simulink model "mikti_sim"  (R2023a)
settings: Solver=ode23tb  StartTime=0.0  StopTime=15  MaxStep=1e-5  MinStep=1e-5  RelTol=1e-4
values from neighbouring files (symbols this model uses):
  A = 0:-1:-50    [mikti.m]
  l = A(i)    [mikti.m]
libraries: spsSeriesRLCBranchLib x9, spsControlledCurrentSourceLib x2, spsCurrentMeasurementLib x2, spsDCVoltageSourceLib x1, spsDCMachineLib x1, spsVoltageMeasurementLib x1, spsControlledVoltageSourceLib x1, sps_lib x1
settings Model: Creator=User  LastModifiedBy=gpapa
settings SolverCC: AlgebraicLoopSolver=TrustRegion
settings DataIOCC: ReturnWorkspaceOutputs=off
settings DebuggingCC: UnconnectedInputMsg=warning  UnconnectedOutputMsg=warning  UnconnectedLineMsg=warning  ArithmeticOperatorsInVariantConditions=warning
settings ModelReferenceCC: EnableRefExpFcnMdlSchedulingChecks=on
settings SFSimCC: CustomCodeUndefinedFunction=UseInterfaceOnly

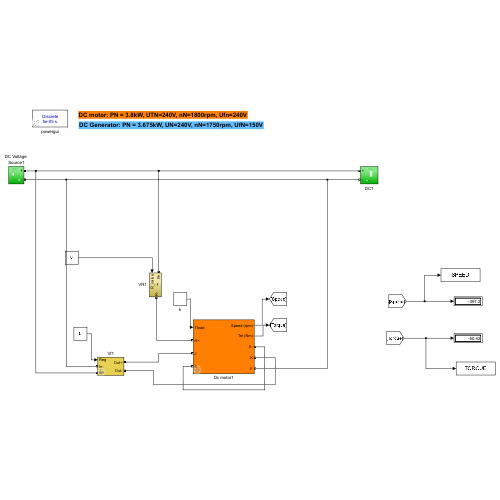
[thumbnail: Simulink's stored preview of the top-level diagram]
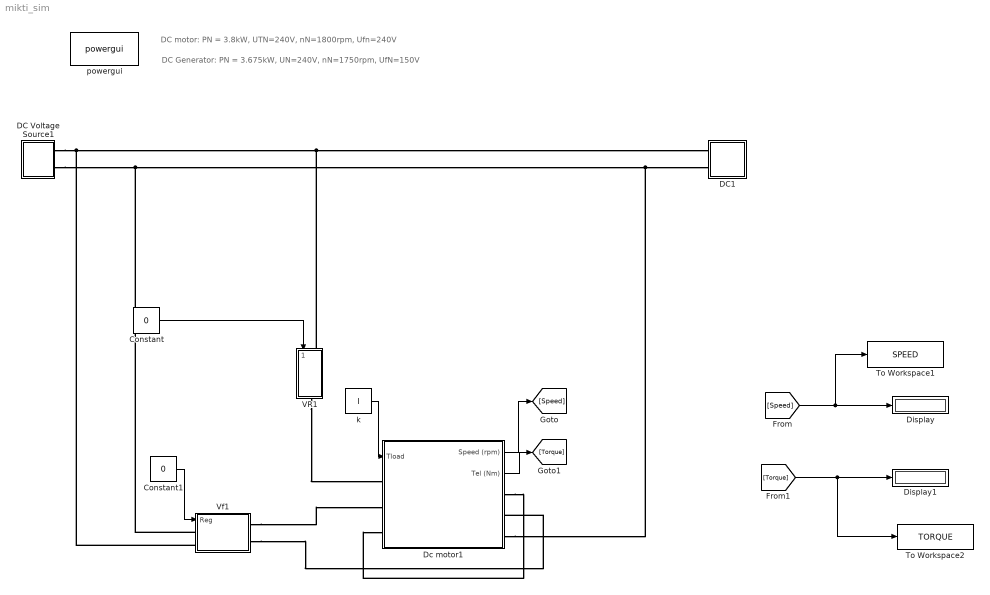
== system mikti_sim ==
  note: DC motor: PN = 3.8kW, UTN=240V, nN=1800rpm, Ufn=240V
  note: DC Generator: PN = 3.675kW, UN=240V, nN=1750rpm, UfN=150V
  Constant : Constant  Value=0
  Constant1 : Constant  Value=0
  DC Voltage Source1 : Subsystem
  DC1 : Subsystem
  Dc motor1 : Subsystem  mask{PN=3.8, VN=240, nN=1800}
      mask prompts: PN "PN (kW)"; VN "VN (V)"; nN "nN (rpm)"
      mask DialogControl Control2 Prompt: DC Motor
  Display : Display
  Display1 : Display
  To Workspace1 : ToWorkspace  VariableName=SPEED  SaveFormat=Structure With Time  SampleTime=-1
      settings: MaxDataPoints=1
  To Workspace2 : ToWorkspace  VariableName=TORQUE  SaveFormat=Structure With Time  SampleTime=-1
      settings: MaxDataPoints=1
  VR1 : Subsystem
  Vf1 : Subsystem  mask{R=230}
      mask prompts: R "R (Ω)"
      mask DialogControl Label1 Prompt: Variable Resistor
  k : Constant  Value=l
  powergui : sps_lib/powergui  Priority=1  SimulationMode=Discrete  SampleTime=50e-6  frequency=60  Iterations=50  frequencyindice=0  Pbase=100e6  ErrMax=1e-4  UnitsV=kV  UnitsW=MW  buscounter=0  FunctionMessages=off  echomessages=off  EnableUseOfTLC=off  CurrentSourceSwitches=off  DisableSnubberDevices=off  DisableRonSwitches=off  DisableVfSwitches=off  DisplayEquations=off  AutomaticDiscreteSolvers=on  SolverType=Tustin/Backward Euler (TBE)  Interpol=off  ExternalGateDelay=off  methode=off  Ts=100  x0status=blocks  SPID=on  SwTol=0  HookPort=off  NonlinearTolerance=1e-4  nMaxIteration=100  ContinueOnMaxIteration=off  RestoreLinks=warning  ResistiveCurrentMeasurement=off  Frange=[0:2:500]  Ylog=off  Xlog=on  ShowGrid=off  save=off  variable=ZData  structure=0  ZoomFFT=off  StartTime=0.0  cycles=1  DisplayStyle=1  fundamental=60  FreqAxis=off  MaxFrequency=1000  frequencyindicesteady=1  RmsSteady=1  display=off
  wires:
  Constant/1 -> VR1/1(R_value)
  Constant1/1 -> Vf1/1(Reg)
  k/1 -> Dc motor1/1(Tload)
  Dc motor1/1(Speed (rpm)) -> [Speed]
  Dc motor1/2(Tel (Nm)) -> [Torque]
  [Speed] -> To Workspace1/1, Display/1
  [Torque] -> To Workspace2/1, Display1/1
  connections:
  DC Voltage Source1/RConn1 -- Vf1/LConn2 -- DC1/LConn1 -- VR1/LConn1
  DC Voltage Source1/RConn2 -- Vf1/LConn1 -- Dc motor1/RConn3 -- DC1/LConn2
  VR1/RConn1 -- Dc motor1/LConn1
  Dc motor1/RConn1 -- Dc motor1/LConn3
  Vf1/RConn1 -- Dc motor1/LConn2
  Vf1/RConn2 -- Dc motor1/RConn2

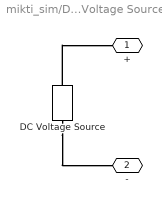
== system mikti_sim/DC Voltage Source1 ==
  DC Voltage Source : spsDCVoltageSourceLib/DC Voltage Source  Amplitude=240  Measurements=None
  + : PMIOPort  Side=Right
  - : PMIOPort  Port=2  Side=Right
  connections:
  DC Voltage Source/LConn1 -- -/RConn1
  DC Voltage Source/RConn1 -- +/RConn1

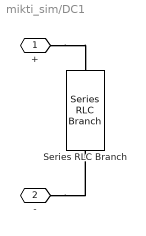
== system mikti_sim/DC1 ==
  Series RLC Branch : spsSeriesRLCBranchLib/Series RLC Branch  LConnTagsString=__new0  RConnTagsString=__new0  BranchType=R  Resistance=1e4  Inductance=1e-3  SetiL0=off  InitialCurrent=0  Capacitance=1e-6  Setx0=off  InitialVoltage=0  Measurements=None
  + : PMIOPort  Side=Left
  - : PMIOPort  Port=2  Side=Left
  connections:
  -/RConn1 -- Series RLC Branch/RConn1
  +/RConn1 -- Series RLC Branch/LConn1

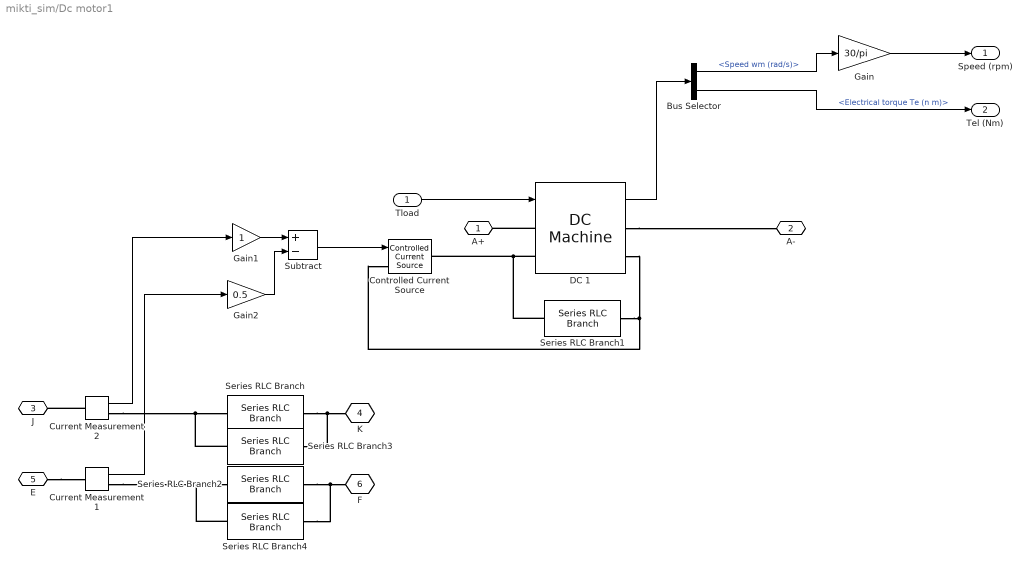
== system mikti_sim/Dc motor1 ==
  Tload : Inport
  Bus Selector : BusSelector  OutputSignals=Speed wm (rad/s),Electrical torque Te (n m)
  Controlled Current Source : spsControlledCurrentSourceLib/Controlled Current Source  Initialize=on  Source_Type=DC  Amplitude=0  Phase=0  Frequency=0  Measurements=None
  Current Measurement1 : spsCurrentMeasurementLib/Current Measurement  PhasorSimulation=off  OutputType=Complex  PSBequivalent=0
  Current Measurement2 : spsCurrentMeasurementLib/Current Measurement  PhasorSimulation=off  OutputType=Complex  PSBequivalent=0
  DC 1 : spsDCMachineLib/DC Machine  PresetModel=No  MechanicalLoad=Torque TL  FieldType=Wound  ShowDetailedParameters=on  MeasurementBus=off  RLa=[0.78 0.016]  RLf=[150 60]  Laf=1.234  MachineConstant=Torque constant (N.m/A)  Ke=1.8  Kt=1.8  J=0.02  Bm=0.01  Tf=0  w0=0  Ifinit=0  TsPowergui=0  TsBlock=-1
  Gain : Gain  Gain=30/pi
  Gain1 : Gain
  Gain2 : Gain  Gain=0.5
  Series RLC Branch : spsSeriesRLCBranchLib/Series RLC Branch  LConnTagsString=__new0  RConnTagsString=__new0  BranchType=RL  Resistance=240  Inductance=120  SetiL0=off  InitialCurrent=0  Capacitance=1e-6  Setx0=off  InitialVoltage=0  Measurements=None
  Series RLC Branch1 : spsSeriesRLCBranchLib/Series RLC Branch  LConnTagsString=__new0  RConnTagsString=__new0  BranchType=R  Resistance=1e6  Inductance=120  SetiL0=off  InitialCurrent=0  Capacitance=1e-6  Setx0=off  InitialVoltage=0  Measurements=None
  Series RLC Branch2 : spsSeriesRLCBranchLib/Series RLC Branch  LConnTagsString=__new0  RConnTagsString=__new0  BranchType=RL  Resistance=0.1  Inductance=1e-3  SetiL0=off  InitialCurrent=0  Capacitance=1e-6  Setx0=off  InitialVoltage=0  Measurements=None
  Series RLC Branch3 : spsSeriesRLCBranchLib/Series RLC Branch  LConnTagsString=__new0  RConnTagsString=__new0  BranchType=R  Resistance=1e6  Inductance=120  SetiL0=off  InitialCurrent=0  Capacitance=1e-6  Setx0=off  InitialVoltage=0  Measurements=None
  Series RLC Branch4 : spsSeriesRLCBranchLib/Series RLC Branch  LConnTagsString=__new0  RConnTagsString=__new0  BranchType=R  Resistance=1e6  Inductance=120  SetiL0=off  InitialCurrent=0  Capacitance=1e-6  Setx0=off  InitialVoltage=0  Measurements=None
  Subtract : Sum  Inputs=+-
  A+ : PMIOPort  Side=Left
  A- : PMIOPort  Port=2  Side=Right
  J : PMIOPort  Port=3  Side=Left
  K : PMIOPort  Port=4  Side=Right
  E : PMIOPort  Port=5  Side=Left
  F : PMIOPort  Port=6  Side=Right
  Speed (rpm) : Outport
  Tel (Nm) : Outport  Port=2
  wires:
  Current Measurement2/1 -> Gain1/1
  Tload/1 -> DC 1/1
  Gain2/1 -> Subtract/2
  Current Measurement1/1 -> Gain2/1
  Subtract/1 -> Controlled Current Source/1
  Gain1/1 -> Subtract/1
  Bus Selector/2 -> Tel (Nm)/1  "<Electrical torque Te (n m)>"
  Gain/1 -> Speed (rpm)/1
  Bus Selector/1 -> Gain/1  "<Speed wm (rad/s)>"
  DC 1/1 -> Bus Selector/1
  connections:
  Series RLC Branch1/RConn1 -- DC 1/RConn2 -- Controlled Current Source/LConn1
  Series RLC Branch1/LConn1 -- DC 1/LConn2 -- Controlled Current Source/RConn1
  Current Measurement2/RConn1 -- Series RLC Branch3/LConn1 -- Series RLC Branch/LConn1
  DC 1/LConn1 -- A+/RConn1
  Current Measurement2/LConn1 -- J/RConn1
  DC 1/RConn1 -- A-/RConn1
  Series RLC Branch/RConn1 -- Series RLC Branch3/RConn1 -- K/RConn1
  E/RConn1 -- Current Measurement1/LConn1
  Current Measurement1/RConn1 -- Series RLC Branch4/LConn1 -- Series RLC Branch2/LConn1
  Series RLC Branch2/RConn1 -- Series RLC Branch4/RConn1 -- F/RConn1

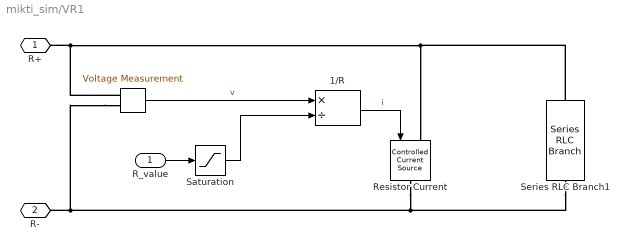
== system mikti_sim/VR1 ==
  R_value : Inport
  " " : spsVoltageMeasurementLib/Voltage Measurement  PhasorSimulation=off  OutputType=Magnitude  PSBequivalent=0
  1/R : Product  Inputs=*/  SaturateOnIntegerOverflow=on  OutDataTypeStr=Inherit: Same as first input
  Resistor Current : spsControlledCurrentSourceLib/Controlled Current Source  Initialize=off  Source_Type=DC  Amplitude=0  Phase=0  Frequency=0  Measurements=None
  Saturation : Saturate  UpperLimit=1e12  LowerLimit=0.01
  Series RLC Branch1 : spsSeriesRLCBranchLib/Series RLC Branch  LConnTagsString=__new0  RConnTagsString=__new0  BranchType=R  Resistance=1e6  Inductance=1e-3  SetiL0=off  InitialCurrent=0  Capacitance=1e-6  Setx0=off  InitialVoltage=0  Measurements=None
  R+ : PMIOPort  Side=Left
  R- : PMIOPort  Port=2  Side=Right
  wires:
  " "/1 -> 1/R/1  "v"
  1/R/1 -> Resistor Current/1  "i"
  R_value/1 -> Saturation/1
  Saturation/1 -> 1/R/2
  connections:
  " "/LConn1 -- Resistor Current/LConn1 -- Series RLC Branch1/LConn1 -- R+/RConn1
  " "/LConn2 -- Series RLC Branch1/RConn1 -- Resistor Current/RConn1 -- R-/RConn1

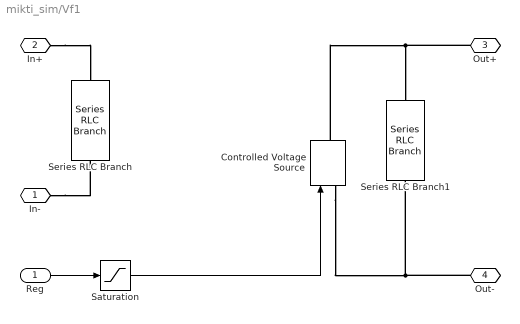
== system mikti_sim/Vf1 ==
  Reg : Inport
  Controlled Voltage Source : spsControlledVoltageSourceLib/Controlled Voltage Source  Initialize=on  Source_Type=DC  Amplitude=0  Phase=0  Frequency=0  Measurements=None
  Saturation : Saturate  UpperLimit=240  LowerLimit=0
  Series RLC Branch : spsSeriesRLCBranchLib/Series RLC Branch  LConnTagsString=__new0  RConnTagsString=__new0  BranchType=R  Resistance=1e6  Inductance=1e-3  SetiL0=off  InitialCurrent=0  Capacitance=1e-6  Setx0=off  InitialVoltage=0  Measurements=None
  Series RLC Branch1 : spsSeriesRLCBranchLib/Series RLC Branch  LConnTagsString=__new0  RConnTagsString=__new0  BranchType=R  Resistance=1e6  Inductance=1e-3  SetiL0=off  InitialCurrent=0  Capacitance=1e-6  Setx0=off  InitialVoltage=0  Measurements=None
  In- : PMIOPort  Side=Left
  In+ : PMIOPort  Port=2  Side=Left
  " Out+" : PMIOPort  Port=3  Side=Right
  " Out-" : PMIOPort  Port=4  Side=Right
  wires:
  Reg/1 -> Saturation/1
  Saturation/1 -> Controlled Voltage Source/1
  connections:
  In+/RConn1 -- Series RLC Branch/LConn1
  In-/RConn1 -- Series RLC Branch/RConn1
  " Out+"/RConn1 -- Controlled Voltage Source/RConn1 -- Series RLC Branch1/LConn1
  " Out-"/RConn1 -- Controlled Voltage Source/LConn1 -- Series RLC Branch1/RConn1
